simulink model "kntl"  (R2025a)
settings: Solver=VariableStepAuto  StartTime=0.0  StopTime=1.0  RelTol=1e-3
values from neighbouring files (symbols this model uses):
  a = (-g + gm)          + gm              * cos(2*pi/p*t_mod+phi0) + j1             * (t_mod.*(t_mod<tE)).^o    [genPoseSynthetic.m]
  D = 2 * zeta * wn * Je    [params.m]
  P = wn^2 * Je    [params.m]    (also in symbolicJacobianSP.m = (R * P.' + t).')
  w_f = wn*5    (= 565.486677646)    [params.m]
undefined symbols (not defined in the file or in its folder): b, w_n
settings Model: Creator=james  LastModifiedBy=james

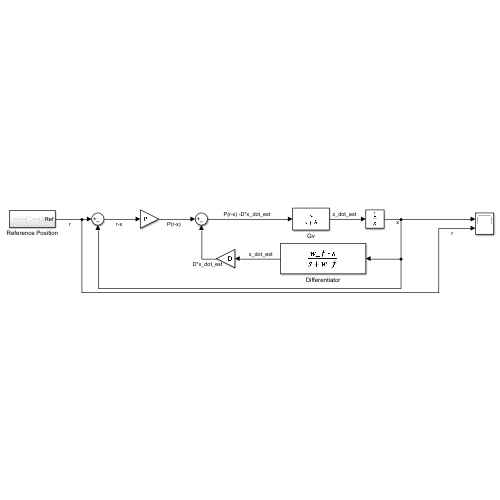
[thumbnail: Simulink's stored preview of the top-level diagram]
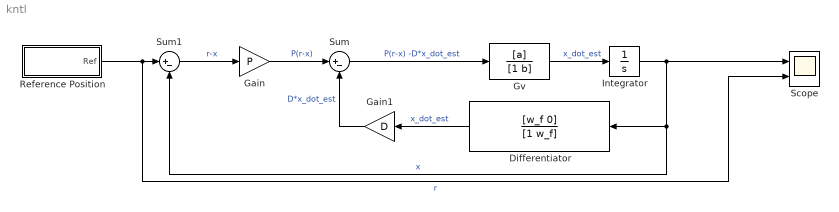
== system kntl ==
  Differentiator : TransferFcn  Numerator=[w_f 0]  Denominator=[1 w_f]
  Gain : Gain  Gain=P
  Gain1 : Gain  Gain=D
  Gv : TransferFcn  Numerator=[a]  Denominator=[1 b]
  Integrator : Integrator
  Reference Position : Subsystem
  Scope : Scope  NumInputPorts=2
      settings: ActiveDisplayYMinimum=-0.011626369102538503  ActiveDisplayYMaximum=0.01273474323576998
  Sum : Sum  Inputs=|+-
  Sum1 : Sum  Inputs=|+-
  wires:
  Reference Position/1(Ref) -> Scope/2, Sum1/1  "r"
  Integrator/1 -> Differentiator/1, Sum1/2, Scope/1  "x"
  Sum1/1 -> Gain/1  "r-x"
  Gain/1 -> Sum/1  "P(r-x)"
  Sum/1 -> Gv/1  "P(r-x) -D*x_dot_est"
  Gain1/1 -> Sum/2  "D*x_dot_est"
  Gv/1 -> Integrator/1  "x_dot_est"
  Differentiator/1 -> Gain1/1  "x_dot_est"

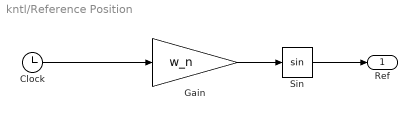
== system kntl/Reference Position ==
  Clock : Clock
  Gain : Gain  Gain=w_n
  Sin : Trigonometry
  Ref : Outport
  wires:
  Clock/1 -> Gain/1
  Sin/1 -> Ref/1
  Gain/1 -> Sin/1
